simulink model "tetha_mu"  (R2022a)
settings: Solver=VariableStepAuto  StartTime=0.0  StopTime=30  RelTol=1e-3
undefined symbols (not defined in the file or in its folder): G_theta_samples
libraries: simulink x4, cstblocks x2
settings Model: Creator=amirhossein  LastModifiedBy=persian
settings SolverCC: AlgebraicLoopSolver=TrustRegion
settings DebuggingCC: UnconnectedInputMsg=warning  UnconnectedOutputMsg=warning  UnconnectedLineMsg=warning  SFMachineParentedDataDiag=warning

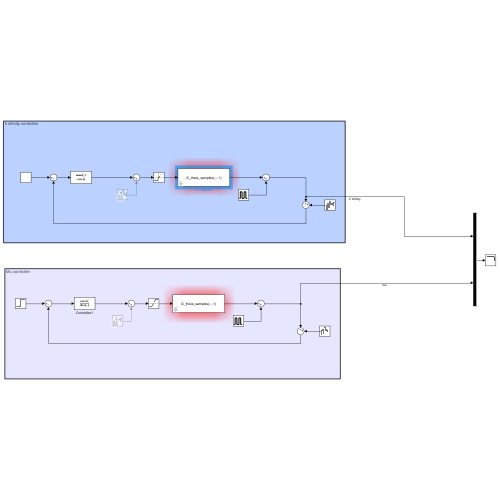
[thumbnail: Simulink's stored preview of the top-level diagram]
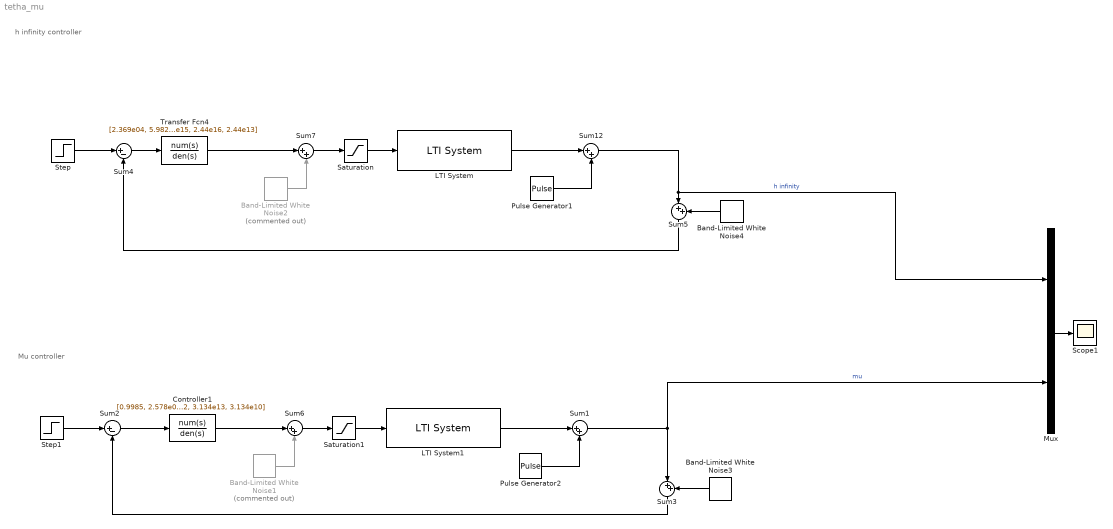
== system tetha_mu ==
  note: Mu controller
  note: h infinity controller
  Band-Limited White Noise1 : simulink/Sources/Band-Limited White Noise  Commented=on  Cov=[0.001]  Ts=0.01  seed=[23341]
  Band-Limited White Noise2 : simulink/Sources/Band-Limited White Noise  Commented=on  Cov=[0.001]  Ts=0.01  seed=[23341]
  Band-Limited White Noise3 : simulink/Sources/Band-Limited White Noise  Cov=[0.0001]  Ts=0.01  seed=[23341]
  Band-Limited White Noise4 : simulink/Sources/Band-Limited White Noise  Cov=[0.0001]  Ts=0.01  seed=[23341]
  Controller1 : TransferFcn  Numerator=[0.9985, 2.578e04, 2.607e07, 1.315e09, 3.189e10, 5.557e11, 4.741e12, 1.34e13]  Denominator=[1, 2.584e04, 2.646e07, 1.678e09, 5.228e10, 8.877e11, 6.458e12, 3.134e13, 3.134e10]
  LTI System : cstblocks/LTI System  sys=G_theta_samples(:,:,1)  IC=[]
  LTI System1 : cstblocks/LTI System  sys=G_theta_samples(:,:,1)  IC=[]
  Mux : Mux  Inputs=2
  Pulse Generator1 : DiscretePulseGenerator  PulseType=Time based  Amplitude=0.1  Period=1.5  PulseWidth=5
  Pulse Generator2 : DiscretePulseGenerator  PulseType=Time based  Amplitude=0.1  Period=1.5  PulseWidth=5
  Saturation : Saturate  UpperLimit=20  LowerLimit=-20
  Saturation1 : Saturate  UpperLimit=20  LowerLimit=-20
  Scope1 : Scope
  Step : Step  SampleTime=0
  Step1 : Step  SampleTime=0
  Sum{1,3,5..7,12} (6 alike) : Sum  Inputs=|++
  Sum2 : Sum  Inputs=|+-
  Sum4 : Sum  Inputs=|+-
  Transfer Fcn4 : TransferFcn  Numerator=[2.369e04, 5.982e08, 2.858e11, 1.872e13, 4.554e14, 8.612e15, 7.941e16, 2.344e17]  Denominator=[1, 2.715e04, 6.056e07, 3.819e10, 3.997e12, 2.164e14, 4.539e15, 2.44e16, 2.44e13]
  wires:
  Mux/1 -> Scope1/1
  Sum5/1 -> Sum4/2
  Sum4/1 -> Transfer Fcn4/1
  Band-Limited White Noise4/1 -> Sum5/2
  Step/1 -> Sum4/1
  Saturation/1 -> LTI System/1
  Sum7/1 -> Saturation/1
  Sum12/1 -> Mux/1, Sum5/1  "h infinity"
  Transfer Fcn4/1 -> Sum7/1
  Band-Limited White Noise2/1 -> Sum7/2
  Pulse Generator1/1 -> Sum12/2
  LTI System/1 -> Sum12/1
  LTI System1/1 -> Sum1/1
  Pulse Generator2/1 -> Sum1/2
  Band-Limited White Noise1/1 -> Sum6/2
  Controller1/1 -> Sum6/1
  Sum1/1 -> Mux/2, Sum3/1  "mu"
  Sum6/1 -> Saturation1/1
  Saturation1/1 -> LTI System1/1
  Step1/1 -> Sum2/1
  Band-Limited White Noise3/1 -> Sum3/2
  Sum2/1 -> Controller1/1
  Sum3/1 -> Sum2/2
